simulink model "forward_velocity_model"  (R2020a)
settings: Solver=VariableStepAuto  StartTime=0.0  StopTime=10.0  RelTol=1e-3
settings Model: Creator=Lord  LastModifiedBy=Lord

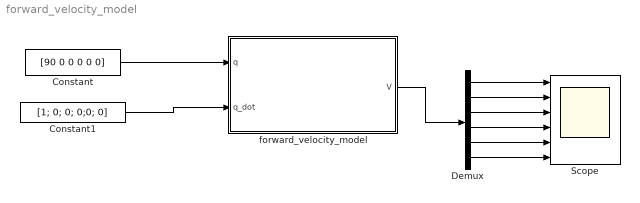
== system forward_velocity_model ==
  Constant : Constant  Value=[90 0 0 0 0 0]
  Constant1 : Constant  Value=[1; 0; 0; 0;0; 0]
  Demux : Demux  Outputs=6
  Scope : Scope  NumInputPorts=6
  forward_velocity_model : MATLAB Function  TreatAsAtomicUnit=on
  wires:
  Constant/1 -> forward_velocity_model/1(q)
  Constant1/1 -> forward_velocity_model/2(q_dot)
  forward_velocity_model/1(V) -> Demux/1
  Demux/1 -> Scope/1
  Demux/2 -> Scope/2
  Demux/3 -> Scope/3
  Demux/4 -> Scope/4
  Demux/5 -> Scope/5
  Demux/6 -> Scope/6

== matlab function forward_velocity_model/forward_velocity_model ==
  data: q input; V output; q_dot input
function V = forward_velocity_model(q,q_dot)

V = zeros(6,1);
j = jacobian_matrix_num(q);
V = j*q_dot;
end
